simulink model "SkywalkerX8_GuidanceAndNavigation_Verification"  (R2018a)
settings: Solver=FixedStepAuto  StartTime=0.0  StopTime=375  FixedStep=0.001  RelTol=1e-3
undefined symbols (not defined in the file): DiscIntNeverNeededParam, F, Light, magnitude, MIL, SkywalkerX8
libraries: simulink_extras x13, sensors x7, simulink x3, sharedTrackingLibrary x2, aerolibwind2 x1, dspmtrx3 x1, dspsigops x1
(part 2 of 3)

== system SkywalkerX8_GuidanceAndNavigation_Verification/Autopilot Digital/Gain Scheduled Controller Phi Digital ==
  note: Since we already essentially have dphi/dt,
      | we can use it directly and create a PIDF controller
      | with PI acting on theta and the "DF" (filtered derivative)
      | simply being a filtered p
  Phi_e : Inport
  Phi : Inport  Port=2
  Va : Inport  Port=3
  p : Inport  Port=4
  DF Controller Phi : Subsystem
  PDF Controller Phi 2DOF : Subsystem
  PDF Controller Phi 2DOF Kd 2D Lookup Table : Lookup_n-D  NumberOfTableDimensions=1  BreakpointsForDimension1=SkywalkerX8.Control.Lateral.SchedulingVariables.VaArray  BreakpointsForDimension2=SkywalkerX8.Control.Longitudinal.SchedulingVariables.alphaArray  Table=SkywalkerX8.Control.Lateral.PhiController.Digital.KdPhi2DOF  InternalRulePriority=Speed  RndMeth=Simplest  InputSameDT=on
  PDF Controller Phi 2DOF Kp 2D Lookup Table : Lookup_n-D  NumberOfTableDimensions=1  BreakpointsForDimension1=SkywalkerX8.Control.Lateral.SchedulingVariables.VaArray  BreakpointsForDimension2=SkywalkerX8.Control.Longitudinal.SchedulingVariables.alphaArray  Table=SkywalkerX8.Control.Lateral.PhiController.Digital.KpPhi2DOF  InternalRulePriority=Speed  RndMeth=Simplest  InputSameDT=on
  PDF Controller Phi 2DOF N 2D Lookup Table : Lookup_n-D  NumberOfTableDimensions=1  BreakpointsForDimension1=SkywalkerX8.Control.Lateral.SchedulingVariables.VaArray  BreakpointsForDimension2=SkywalkerX8.Control.Longitudinal.SchedulingVariables.alphaArray  Table=SkywalkerX8.Control.Lateral.PhiController.Digital.NPhi2DOF  InternalRulePriority=Speed  RndMeth=Simplest  InputSameDT=on
  PI Controller Phi : Subsystem
  PIDF Controller Phi Kd 2D Lookup Table : Lookup_n-D  NumberOfTableDimensions=1  BreakpointsForDimension1=SkywalkerX8.Control.Lateral.SchedulingVariables.VaArray  BreakpointsForDimension2=SkywalkerX8.Control.Longitudinal.SchedulingVariables.alphaArray  Table=SkywalkerX8.Control.Lateral.PhiController.Digital.KdPhi  InternalRulePriority=Speed  RndMeth=Simplest  InputSameDT=on
  PIDF Controller Phi Ki 2D Lookup Table : Lookup_n-D  NumberOfTableDimensions=1  BreakpointsForDimension1=SkywalkerX8.Control.Lateral.SchedulingVariables.VaArray  BreakpointsForDimension2=SkywalkerX8.Control.Longitudinal.SchedulingVariables.alphaArray  Table=SkywalkerX8.Control.Lateral.PhiController.Digital.KiPhi  InternalRulePriority=Speed  RndMeth=Simplest  InputSameDT=on
  PIDF Controller Phi Kp 2D Lookup Table : Lookup_n-D  NumberOfTableDimensions=1  BreakpointsForDimension1=SkywalkerX8.Control.Lateral.SchedulingVariables.VaArray  BreakpointsForDimension2=SkywalkerX8.Control.Longitudinal.SchedulingVariables.alphaArray  Table=SkywalkerX8.Control.Lateral.PhiController.Digital.KpPhi  InternalRulePriority=Speed  RndMeth=Simplest  InputSameDT=on
  PIDF Controller Phi N 2D Lookup Table : Lookup_n-D  NumberOfTableDimensions=1  BreakpointsForDimension1=SkywalkerX8.Control.Lateral.SchedulingVariables.VaArray  BreakpointsForDimension2=SkywalkerX8.Control.Longitudinal.SchedulingVariables.alphaArray  Table=SkywalkerX8.Control.Lateral.PhiController.Digital.NPhi  InternalRulePriority=Speed  RndMeth=Simplest  InputSameDT=on
  Saturation : Saturate  UpperLimit=SkywalkerX8.Control.Lateral.PhiController.upperSaturationDa  LowerLimit=SkywalkerX8.Control.Lateral.PhiController.lowerSaturationDa
  Sum1 : Sum  Inputs=+++|
  Zero-Order Hold : ZeroOrderHold  SampleTime=SkywalkerX8.Control.Lateral.PhiController.Digital.SampleTime
  da : Outport
  wires:
  Va/1 -> PDF Controller Phi 2DOF Kp 2D Lookup Table/1, PDF Controller Phi 2DOF Kd 2D Lookup Table/1, PDF Controller Phi 2DOF N 2D Lookup Table/1, PIDF Controller Phi N 2D Lookup Table/1, PIDF Controller Phi Kd 2D Lookup Table/1, PIDF Controller Phi Ki 2D Lookup Table/1, PIDF Controller Phi Kp 2D Lookup Table/1
  Phi_e/1 -> PI Controller Phi/1(u)
  PIDF Controller Phi Kp 2D Lookup Table/1 -> PI Controller Phi/2(P)
  PIDF Controller Phi Ki 2D Lookup Table/1 -> PI Controller Phi/3(I)
  PI Controller Phi/1(y) -> Sum1/2
  Sum1/1 -> Saturation/1, PI Controller Phi/5(Pre-Saturation)
  p/1 -> DF Controller Phi/3(du/dt)
  DF Controller Phi/1(da*) -> Sum1/3
  PIDF Controller Phi N 2D Lookup Table/1 -> DF Controller Phi/1(N)
  PIDF Controller Phi Kd 2D Lookup Table/1 -> DF Controller Phi/2(D)
  Saturation/1 -> Zero-Order Hold/1, PI Controller Phi/4(Post-Saturation)
  PDF Controller Phi 2DOF Kp 2D Lookup Table/1 -> PDF Controller Phi 2DOF/2(P)
  PDF Controller Phi 2DOF Kd 2D Lookup Table/1 -> PDF Controller Phi 2DOF/3(D)
  PDF Controller Phi 2DOF N 2D Lookup Table/1 -> PDF Controller Phi 2DOF/4(N)
  Phi/1 -> PDF Controller Phi 2DOF/1(u)
  PDF Controller Phi 2DOF/1(y) -> Sum1/1
  Zero-Order Hold/1 -> da/1

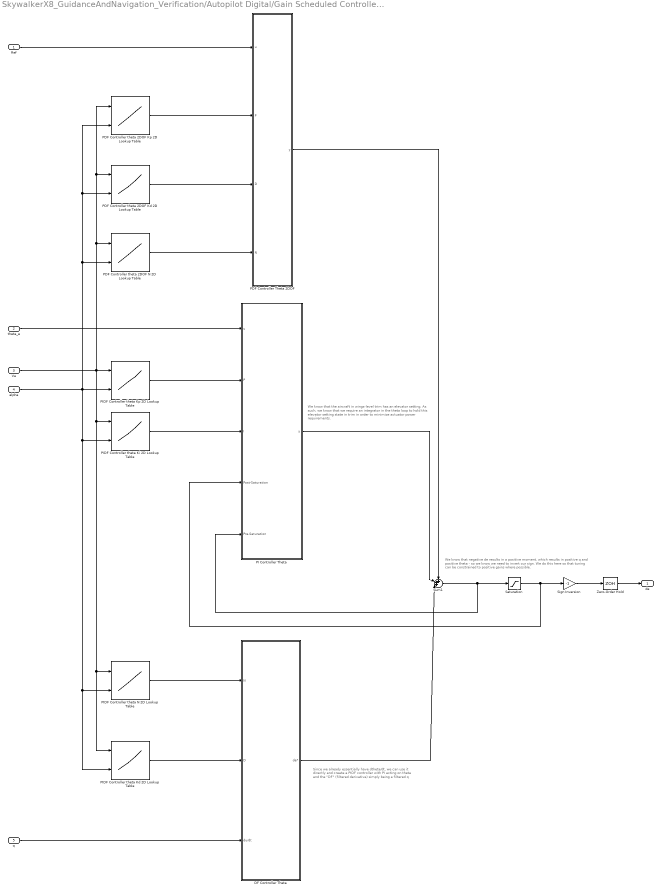
== system SkywalkerX8_GuidanceAndNavigation_Verification/Autopilot Digital/Gain Scheduled Controller Theta Digital ==
  note: Since we already essentially have dtheta/dt,
      | we can use it directly and create a PIDF controller
      | with PI acting on theta and the "DF" (filtered derivative)
      | simply being a filtered q
  note: We know that negative de results in a positive moment, which results in
      | positive q and positive theta - so we know we need to invert our sign.
      | We do this here so that tuning can be constrained to positive gains where possible.
  note: We know that the aircraft in wings-level trim has an elevator setting. As such, we know that we require an integrator in the theta loop to hold this elevator setting state in trim in order to minimize actuator power requirements.
  Ref : Inport
  theta_e : Inport  Port=2
  Va : Inport  Port=3
  alpha : Inport  Port=4
  q : Inport  Port=5
  DF Controller Theta : Subsystem
  PDF Controller Theta 2DOF : Subsystem
  PDF Controller theta 2DOF Kd 2D Lookup Table : Lookup_n-D  BreakpointsForDimension1=SkywalkerX8.Control.Longitudinal.SchedulingVariables.VaArray  BreakpointsForDimension2=SkywalkerX8.Control.Longitudinal.SchedulingVariables.alphaArray  BeginIndexSearchUsingPreviousIndexResult=on  Table=SkywalkerX8.Control.Longitudinal.thetaController.Digital.KdTheta2DOF  InternalRulePriority=Speed  RndMeth=Simplest  InputSameDT=on
  PDF Controller theta 2DOF Kp 2D Lookup Table : Lookup_n-D  BreakpointsForDimension1=SkywalkerX8.Control.Longitudinal.SchedulingVariables.VaArray  BreakpointsForDimension2=SkywalkerX8.Control.Longitudinal.SchedulingVariables.alphaArray  Table=SkywalkerX8.Control.Longitudinal.thetaController.Digital.KpTheta2DOF  InternalRulePriority=Speed  RndMeth=Simplest  InputSameDT=on
  PDF Controller theta 2DOF N 2D Lookup Table : Lookup_n-D  BreakpointsForDimension1=SkywalkerX8.Control.Longitudinal.SchedulingVariables.VaArray  BreakpointsForDimension2=SkywalkerX8.Control.Longitudinal.SchedulingVariables.alphaArray  Table=SkywalkerX8.Control.Longitudinal.thetaController.Digital.NTheta2DOF  InternalRulePriority=Speed  RndMeth=Simplest  InputSameDT=on
  PI Controller Theta : Subsystem
  PIDF Controller theta Kd 2D Lookup Table : Lookup_n-D  BreakpointsForDimension1=SkywalkerX8.Control.Longitudinal.SchedulingVariables.VaArray  BreakpointsForDimension2=SkywalkerX8.Control.Longitudinal.SchedulingVariables.alphaArray  Table=SkywalkerX8.Control.Longitudinal.thetaController.Digital.KdTheta  InternalRulePriority=Speed  RndMeth=Simplest  InputSameDT=on
  PIDF Controller theta Ki 2D Lookup Table : Lookup_n-D  BreakpointsForDimension1=SkywalkerX8.Control.Longitudinal.SchedulingVariables.VaArray  BreakpointsForDimension2=SkywalkerX8.Control.Longitudinal.SchedulingVariables.alphaArray  Table=SkywalkerX8.Control.Longitudinal.thetaController.Digital.KiTheta  InternalRulePriority=Speed  RndMeth=Simplest  InputSameDT=on
  PIDF Controller theta Kp 2D Lookup Table : Lookup_n-D  BreakpointsForDimension1=SkywalkerX8.Control.Longitudinal.SchedulingVariables.VaArray  BreakpointsForDimension2=SkywalkerX8.Control.Longitudinal.SchedulingVariables.alphaArray  Table=SkywalkerX8.Control.Longitudinal.thetaController.Digital.KpTheta  InternalRulePriority=Speed  RndMeth=Simplest  InputSameDT=on
  PIDF Controller theta N 2D Lookup Table : Lookup_n-D  BreakpointsForDimension1=SkywalkerX8.Control.Longitudinal.SchedulingVariables.VaArray  BreakpointsForDimension2=SkywalkerX8.Control.Longitudinal.SchedulingVariables.alphaArray  Table=SkywalkerX8.Control.Longitudinal.thetaController.Digital.NTheta  InternalRulePriority=Speed  RndMeth=Simplest  InputSameDT=on
  Saturation : Saturate  UpperLimit=SkywalkerX8.Control.Longitudinal.thetaController.Digital.upperSaturationNegativeDe  LowerLimit=SkywalkerX8.Control.Longitudinal.thetaController.Digital.lowerSaturationNegativeDe
  Sign Inversion : Gain  Gain=-1
  Sum1 : Sum  Inputs=+++|
  Zero-Order Hold : ZeroOrderHold  SampleTime=SkywalkerX8.Control.Longitudinal.thetaController.Digital.SampleTime
  de : Outport
  wires:
  Va/1 -> PDF Controller theta 2DOF Kd 2D Lookup Table/1, PDF Controller theta 2DOF Kp 2D Lookup Table/1, PDF Controller theta 2DOF N 2D Lookup Table/1, PIDF Controller theta N 2D Lookup Table/1, PIDF Controller theta Kd 2D Lookup Table/1, PIDF Controller theta Ki 2D Lookup Table/1, PIDF Controller theta Kp 2D Lookup Table/1
  theta_e/1 -> PI Controller Theta/1(u)
  PIDF Controller theta Kp 2D Lookup Table/1 -> PI Controller Theta/2(P)
  PIDF Controller theta Ki 2D Lookup Table/1 -> PI Controller Theta/3(I)
  alpha/1 -> PDF Controller theta 2DOF N 2D Lookup Table/2, PDF Controller theta 2DOF Kd 2D Lookup Table/2, PDF Controller theta 2DOF Kp 2D Lookup Table/2, PIDF Controller theta N 2D Lookup Table/2, PIDF Controller theta Kd 2D Lookup Table/2, PIDF Controller theta Ki 2D Lookup Table/2, PIDF Controller theta Kp 2D Lookup Table/2
  PI Controller Theta/1(y) -> Sum1/2
  Sum1/1 -> Saturation/1, PI Controller Theta/5(Pre-Saturation)
  Saturation/1 -> Sign Inversion/1, PI Controller Theta/4(Post-Saturation)
  PIDF Controller theta N 2D Lookup Table/1 -> DF Controller Theta/1(N)
  PIDF Controller theta Kd 2D Lookup Table/1 -> DF Controller Theta/2(D)
  q/1 -> DF Controller Theta/3(du/dt)
  DF Controller Theta/1(de*) -> Sum1/3
  Sign Inversion/1 -> Zero-Order Hold/1
  PDF Controller theta 2DOF Kp 2D Lookup Table/1 -> PDF Controller Theta 2DOF/2(P)
  PDF Controller theta 2DOF Kd 2D Lookup Table/1 -> PDF Controller Theta 2DOF/3(D)
  PDF Controller theta 2DOF N 2D Lookup Table/1 -> PDF Controller Theta 2DOF/4(N)
  Ref/1 -> PDF Controller Theta 2DOF/1(u)
  PDF Controller Theta 2DOF/1(y) -> Sum1/1
  Zero-Order Hold/1 -> de/1

== system SkywalkerX8_GuidanceAndNavigation_Verification/Autopilot Digital/Gain Scheduled Controller Va_dt Digital ==
  Va_e : Inport
  Va : Inport  Port=2
  TR : Inport  Port=3
  PIDF Controller Va_dt : Subsystem
  PIDF Controller Va_dt Kd Lookup Table : Lookup_n-D  NumberOfTableDimensions=1  BreakpointsForDimension1=SkywalkerX8.Control.Longitudinal.SchedulingVariables.VaArray  BreakpointsForDimension2=[1 2 3 4 5]  Table=SkywalkerX8.Control.Longitudinal.VaDtController.Digital.KdVaDt  InternalRulePriority=Speed  RndMeth=Simplest  InputSameDT=on
  PIDF Controller Va_dt Ki Lookup Table : Lookup_n-D  NumberOfTableDimensions=1  BreakpointsForDimension1=SkywalkerX8.Control.Longitudinal.SchedulingVariables.VaArray  BreakpointsForDimension2=[1 2 3 4 5]  Table=SkywalkerX8.Control.Longitudinal.VaDtController.Digital.KiVaDt  InternalRulePriority=Speed  RndMeth=Simplest  InputSameDT=on
  PIDF Controller Va_dt Kp Lookup Table : Lookup_n-D  NumberOfTableDimensions=1  BreakpointsForDimension1=SkywalkerX8.Control.Longitudinal.SchedulingVariables.VaArray  BreakpointsForDimension2=[1 2 3 4 5]  Table=SkywalkerX8.Control.Longitudinal.VaDtController.Digital.KpVaDt  InternalRulePriority=Speed  RndMeth=Simplest  InputSameDT=on
  PIDF Controller Va_dt Kt Tracking Gain Scalar : Gain  Gain=SkywalkerX8.Control.Longitudinal.VaDtController.KtScalar
  PIDF Controller Va_dt N Lookup Table : Lookup_n-D  NumberOfTableDimensions=1  BreakpointsForDimension1=SkywalkerX8.Control.Longitudinal.SchedulingVariables.VaArray  BreakpointsForDimension2=[1 2 3 4 5]  Table=SkywalkerX8.Control.Longitudinal.VaDtController.Digital.NVaDt  InternalRulePriority=Speed  RndMeth=Simplest  InputSameDT=on
  Zero-Order Hold : ZeroOrderHold  SampleTime=SkywalkerX8.Control.Longitudinal.VaDtController.Digital.SampleTime
  dt : Outport
  wires:
  Va_e/1 -> PIDF Controller Va_dt/1(u)
  PIDF Controller Va_dt/1(y) -> Zero-Order Hold/1
  PIDF Controller Va_dt Kp Lookup Table/1 -> PIDF Controller Va_dt/2(P)
  Va/1 -> PIDF Controller Va_dt Kp Lookup Table/1, PIDF Controller Va_dt Ki Lookup Table/1, PIDF Controller Va_dt N Lookup Table/1, PIDF Controller Va_dt Kd Lookup Table/1
  PIDF Controller Va_dt Ki Lookup Table/1 -> PIDF Controller Va_dt/3(I), PIDF Controller Va_dt Kt Tracking Gain Scalar/1
  PIDF Controller Va_dt Kd Lookup Table/1 -> PIDF Controller Va_dt/4(D)
  PIDF Controller Va_dt N Lookup Table/1 -> PIDF Controller Va_dt/5(N)
  TR/1 -> PIDF Controller Va_dt/7(TR)
  PIDF Controller Va_dt Kt Tracking Gain Scalar/1 -> PIDF Controller Va_dt/6(Kt)
  Zero-Order Hold/1 -> dt/1

== system SkywalkerX8_GuidanceAndNavigation_Verification/Autopilot Digital/Gain Scheduled Controller Va_theta Digital ==
  note: We know that negative theta results in positive Va (as we'll start losing altitude)
      | and vice versa as we gain altitude. In order to keep our controller gains positive
      |  we do the sign inversion seperately.
  note: Because we sign invert the output, we need to sign invert the tracking
      | value
  Va_e : Inport
  Va : Inport  Port=2
  alpha : Inport  Port=3
  TR : Inport  Port=4
  PIDF Controller Va_theta : Subsystem
  PIDF Controller Va_theta Kd 2D Lookup Table : Lookup_n-D  BreakpointsForDimension1=SkywalkerX8.Control.Longitudinal.SchedulingVariables.VaArray  BreakpointsForDimension2=SkywalkerX8.Control.Longitudinal.SchedulingVariables.alphaArray  Table=SkywalkerX8.Control.Longitudinal.VaThetaController.Digital.KdVaTheta  InternalRulePriority=Speed  RndMeth=Simplest  InputSameDT=on
  PIDF Controller Va_theta Ki 2D Lookup Table : Lookup_n-D  BreakpointsForDimension1=SkywalkerX8.Control.Longitudinal.SchedulingVariables.VaArray  BreakpointsForDimension2=SkywalkerX8.Control.Longitudinal.SchedulingVariables.alphaArray  Table=SkywalkerX8.Control.Longitudinal.VaThetaController.Digital.KiVaTheta  InternalRulePriority=Speed  RndMeth=Simplest  InputSameDT=on
  PIDF Controller Va_theta Kp 2D Lookup Table : Lookup_n-D  BreakpointsForDimension1=SkywalkerX8.Control.Longitudinal.SchedulingVariables.VaArray  BreakpointsForDimension2=SkywalkerX8.Control.Longitudinal.SchedulingVariables.alphaArray  Table=SkywalkerX8.Control.Longitudinal.VaThetaController.Digital.KpVaTheta  InternalRulePriority=Speed  RndMeth=Simplest  InputSameDT=on
  PIDF Controller Va_theta Kt Tracking Gain Scalar : Gain  Gain=SkywalkerX8.Control.Longitudinal.VaThetaController.KtScalar
  PIDF Controller Va_theta N 2D Lookup Table : Lookup_n-D  BreakpointsForDimension1=SkywalkerX8.Control.Longitudinal.SchedulingVariables.VaArray  BreakpointsForDimension2=SkywalkerX8.Control.Longitudinal.SchedulingVariables.alphaArray  Table=SkywalkerX8.Control.Longitudinal.VaThetaController.Digital.NVaTheta  InternalRulePriority=Speed  RndMeth=Simplest  InputSameDT=on
  Sign Inversion : Gain  Gain=-1
  Tracking Sign Inversion : Gain  Gain=-1
  Zero-Order Hold : ZeroOrderHold  SampleTime=SkywalkerX8.Control.Longitudinal.altController.Digital.SampleTime
  theta_c_Va : Outport
  wires:
  Va_e/1 -> PIDF Controller Va_theta/1(u)
  PIDF Controller Va_theta/1(y) -> Sign Inversion/1
  PIDF Controller Va_theta Kp 2D Lookup Table/1 -> PIDF Controller Va_theta/2(P)
  Va/1 -> PIDF Controller Va_theta Kp 2D Lookup Table/1, PIDF Controller Va_theta Ki 2D Lookup Table/1, PIDF Controller Va_theta N 2D Lookup Table/1, PIDF Controller Va_theta Kd 2D Lookup Table/1
  PIDF Controller Va_theta Ki 2D Lookup Table/1 -> PIDF Controller Va_theta/3(I), PIDF Controller Va_theta Kt Tracking Gain Scalar/1
  PIDF Controller Va_theta Kd 2D Lookup Table/1 -> PIDF Controller Va_theta/4(D)
  PIDF Controller Va_theta N 2D Lookup Table/1 -> PIDF Controller Va_theta/5(N)
  alpha/1 -> PIDF Controller Va_theta Kp 2D Lookup Table/2, PIDF Controller Va_theta Ki 2D Lookup Table/2, PIDF Controller Va_theta N 2D Lookup Table/2, PIDF Controller Va_theta Kd 2D Lookup Table/2
  Sign Inversion/1 -> Zero-Order Hold/1
  TR/1 -> Tracking Sign Inversion/1
  PIDF Controller Va_theta Kt Tracking Gain Scalar/1 -> PIDF Controller Va_theta/6(Kt)
  Tracking Sign Inversion/1 -> PIDF Controller Va_theta/7(TR)
  Zero-Order Hold/1 -> theta_c_Va/1

== system SkywalkerX8_GuidanceAndNavigation_Verification/Autopilot Digital/Gain Scheduled Controller h_theta Digital ==
  note: We know that wings-level trim has the aircraft with a pitch angle. As such,
      | we know that at a minimum this controller has to be a PI controller, because otherwise
      | we have no state to hold the required steady state theta command.
  h_e : Inport
  TR : Inport  Port=2
  Kd : Constant  Value=SkywalkerX8.Control.Longitudinal.altController.Digital.KdAlt(5, 3)
  Ki : Constant  Value=SkywalkerX8.Control.Longitudinal.altController.Digital.KiAlt(5, 3)
  Kp : Constant  Value=SkywalkerX8.Control.Longitudinal.altController.Digital.KpAlt(5, 3)
  Kt : Constant  Value=SkywalkerX8.Control.Longitudinal.altController.KtScalar*SkywalkerX8.Control.Longitudinal.altController.Digital.KiAlt(5, 3)
  N : Constant  Value=SkywalkerX8.Control.Longitudinal.altController.Digital.NAlt(5, 3)
  PIDF Controller h_theta : Subsystem
  Zero-Order Hold : ZeroOrderHold  SampleTime=SkywalkerX8.Control.Longitudinal.altController.Digital.SampleTime
  theta_c_h : Outport
  wires:
  Kp/1 -> PIDF Controller h_theta/2(P)
  h_e/1 -> PIDF Controller h_theta/1(u)
  Kd/1 -> PIDF Controller h_theta/4(D)
  N/1 -> PIDF Controller h_theta/5(N)
  PIDF Controller h_theta/1(y) -> Zero-Order Hold/1
  TR/1 -> PIDF Controller h_theta/7(TR)
  Ki/1 -> PIDF Controller h_theta/3(I)
  Kt/1 -> PIDF Controller h_theta/6(Kt)
  Zero-Order Hold/1 -> theta_c_h/1

== system SkywalkerX8_GuidanceAndNavigation_Verification/Autopilot Digital/h Rate Limiter Dynamic ==
  note: U(k)
  note: Y(k)
  up : Inport
  u : Inport  Port=2
  lo : Inport  Port=3
  Delay Input2 : UnitDelay  Description=Store in Global RAM  DisableCoverage=on  InitialCondition=initOutput  SampleTime=-1
  Difference Inputs1 : Sum  Description=Add in CPU  DisableCoverage=on  Inputs=+-  OutDataTypeStr=Inherit: Inherit via back propagation
  Difference Inputs2 : Sum  Description=Add in CPU  OutDataTypeStr=Inherit: Inherit via back propagation
  FixPt Data Type Duplicate : DataTypeDuplicate  DisableCoverage=on  NumInputPorts=7
  Saturation Dynamic : simulink/Discontinuities/Saturation Dynamic  OutMin=[]  OutMax=[]  OutDataTypeStr=Inherit: Same as second input  OutDataType=fixdt(1, 16)  OutScaling=2^-10  DoSatur=off
  delta fall limit : Product  DisableCoverage=on  Inputs=**  OutDataTypeStr=Inherit: Inherit via back propagation  SaturateOnIntegerOverflow=on
  delta rise limit : Product  DisableCoverage=on  Inputs=**  OutDataTypeStr=Inherit: Inherit via back propagation  SaturateOnIntegerOverflow=on
  sample time : SampleTimeMath  DisableCoverage=on  TsampMathOp=Ts Only  weightValue=1
  Y : Outport  InitialOutput=0
  wires:
  Delay Input2/1 -> Difference Inputs1/2, FixPt Data Type Duplicate/2, Difference Inputs2/2  "Y(k-1)"
  Difference Inputs1/1 -> FixPt Data Type Duplicate/4, Saturation Dynamic/2  "( U(k) - Y(k-1) )"
  Difference Inputs2/1 -> Y/1, Delay Input2/1, FixPt Data Type Duplicate/1
  u/1 -> Difference Inputs1/1, FixPt Data Type Duplicate/5, sample time/1
  delta fall limit/1 -> FixPt Data Type Duplicate/3, Saturation Dynamic/3
  sample time/1 -> delta fall limit/2, delta rise limit/2
  Saturation Dynamic/1 -> Difference Inputs2/1, FixPt Data Type Duplicate/7
  delta rise limit/1 -> FixPt Data Type Duplicate/6, Saturation Dynamic/1
  lo/1 -> delta fall limit/1
  up/1 -> delta rise limit/1

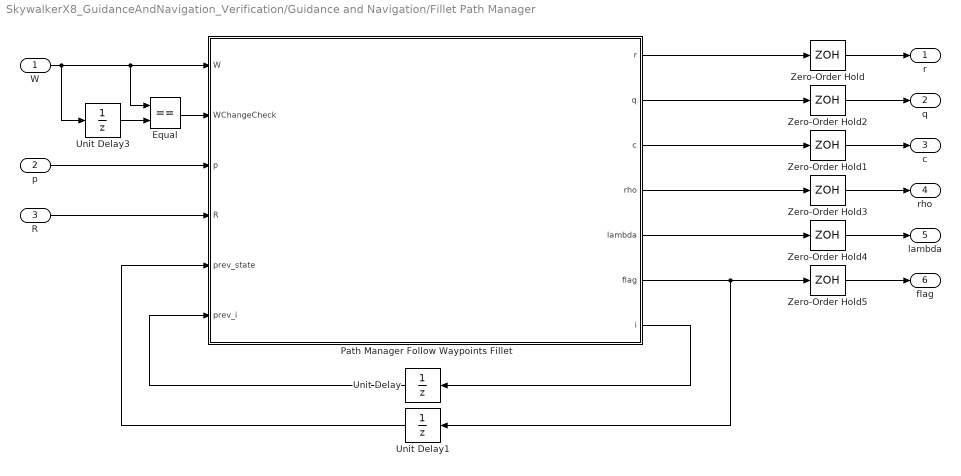
== system SkywalkerX8_GuidanceAndNavigation_Verification/Guidance and Navigation/Fillet Path Manager ==
  W : Inport
  p : Inport  Port=2
  R : Inport  Port=3
  Equal : RelationalOperator  Operator===  OutDataTypeStr=boolean  RndMeth=Simplest
  Path Manager Follow Waypoints Fillet : MATLAB Function  TreatAsAtomicUnit=on
  Unit Delay : UnitDelay  InitialCondition=2  SampleTime=SampleTime
  Unit Delay1 : UnitDelay  InitialCondition=1  SampleTime=SampleTime
  Unit Delay3 : UnitDelay  InitialCondition=SkywalkerX8.Test.Waypoints  SampleTime=SampleTime
  Zero-Order Hold{,1..5} (6 alike) : ZeroOrderHold  SampleTime=SampleTime
  r : Outport
  q : Outport  Port=2
  c : Outport  Port=3
  rho : Outport  Port=4
  lambda : Outport  Port=5
  flag : Outport  Port=6
  wires:
  Path Manager Follow Waypoints Fillet/2(q) -> Zero-Order Hold2/1
  Path Manager Follow Waypoints Fillet/6(flag) -> Zero-Order Hold5/1, Unit Delay1/1
  W/1 -> Unit Delay3/1, Equal/1, Path Manager Follow Waypoints Fillet/1(W)
  Unit Delay/1 -> Path Manager Follow Waypoints Fillet/6(prev_i)
  Path Manager Follow Waypoints Fillet/7(i) -> Unit Delay/1
  Path Manager Follow Waypoints Fillet/3(c) -> Zero-Order Hold1/1
  p/1 -> Path Manager Follow Waypoints Fillet/3(p)
  Path Manager Follow Waypoints Fillet/4(rho) -> Zero-Order Hold3/1
  Path Manager Follow Waypoints Fillet/1(r) -> Zero-Order Hold/1
  Unit Delay1/1 -> Path Manager Follow Waypoints Fillet/5(prev_state)
  R/1 -> Path Manager Follow Waypoints Fillet/4(R)
  Zero-Order Hold/1 -> r/1
  Zero-Order Hold1/1 -> c/1
  Zero-Order Hold2/1 -> q/1
  Zero-Order Hold3/1 -> rho/1
  Zero-Order Hold4/1 -> lambda/1
  Zero-Order Hold5/1 -> flag/1
  Path Manager Follow Waypoints Fillet/5(lambda) -> Zero-Order Hold4/1
  Unit Delay3/1 -> Equal/2
  Equal/1 -> Path Manager Follow Waypoints Fillet/2(WChangeCheck)

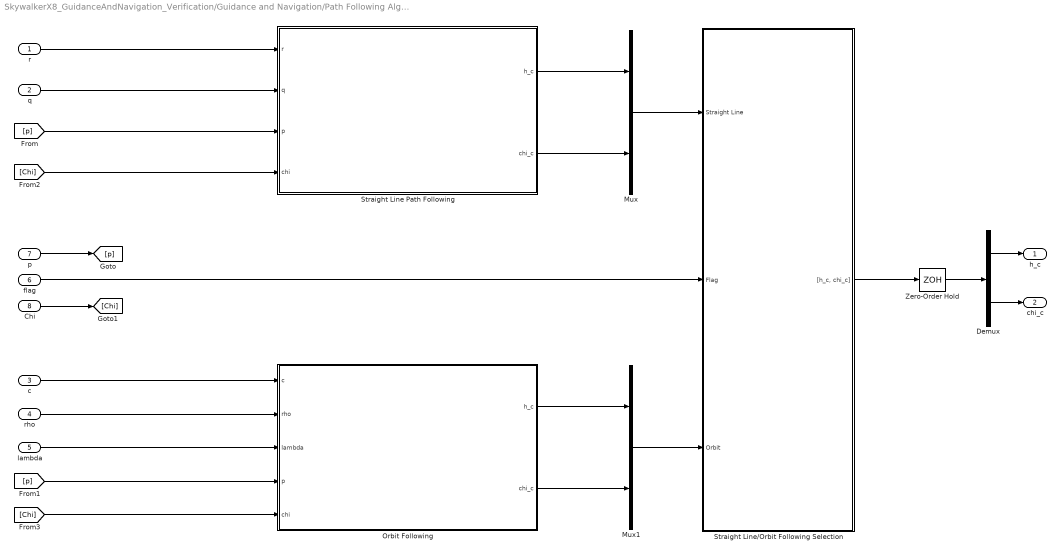
== system SkywalkerX8_GuidanceAndNavigation_Verification/Guidance and Navigation/Path Following Algorithm ==
  r : Inport
  q : Inport  Port=2
  c : Inport  Port=3
  rho : Inport  Port=4
  lambda : Inport  Port=5
  flag : Inport  Port=6
  p : Inport  Port=7
  Chi : Inport  Port=8
  Demux : Demux  Outputs=2
  Mux : Mux  Inputs=2
  Mux1 : Mux  Inputs=2
  Orbit Following : MATLAB Function  TreatAsAtomicUnit=on  mask{korbit=korbit}
      mask prompts: korbit "kOrbit (Unitless)"
  Straight Line Path Following : MATLAB Function  TreatAsAtomicUnit=on  mask{chi_inf=ChiInf, kpath=kpath}
      mask prompts: chi_inf "Chi_inf (rad)"; kpath "kPath (Unitless)"
  Straight Line/Orbit Following Selection : Subsystem
      mask Display:
      | port_label('input', 1, '[h_c, \chi_c]_{Straight Line} (m, rad)', 'texMode', 'On')
      | port_label('input', 2, 'Flag (Unitless)', 'texMode', 'On')
      | port_label('input', 3, '[h_c, \chi_c]_{Orbit Following} (m, rad)', 'texMode', 'On')
      | 
      | port_label('output', 1, '[h_c, \chi_c] (m, rad)', 'texMode', 'On')
  Zero-Order Hold : ZeroOrderHold  SampleTime=SampleTime
  h_c : Outport
  chi_c : Outport  Port=2
  wires:
  [Chi] -> Orbit Following/5(chi)
  rho/1 -> Orbit Following/2(rho)
  r/1 -> Straight Line Path Following/1(r)
  Orbit Following/2(chi_c) -> Mux1/2
  q/1 -> Straight Line Path Following/2(q)
  p/1 -> [p]
  lambda/1 -> Orbit Following/3(lambda)
  Orbit Following/1(h_c) -> Mux1/1
  Straight Line/Orbit Following Selection/1("[h_c, chi_c]") -> Zero-Order Hold/1
  Mux/1 -> Straight Line/Orbit Following Selection/1(Straight Line)
  c/1 -> Orbit Following/1(c)
  Mux1/1 -> Straight Line/Orbit Following Selection/3(Orbit)
  Straight Line Path Following/2(chi_c) -> Mux/2
  [Chi] -> Straight Line Path Following/4(chi)
  flag/1 -> Straight Line/Orbit Following Selection/2(Flag)
  [p] -> Straight Line Path Following/3(p)
  Straight Line Path Following/1(h_c) -> Mux/1
  Chi/1 -> [Chi]
  [p] -> Orbit Following/4(p)
  Zero-Order Hold/1 -> Demux/1
  Demux/1 -> h_c/1
  Demux/2 -> chi_c/1

== system SkywalkerX8_GuidanceAndNavigation_Verification/Sensor Suite/9-Axis MEMS IMU ==
  ainertial : Inport
  PhiThetaPsi : Inport  Port=2
  pqr : Inport  Port=3
  3-Axis Accelerometer : sensors/3-Axis Accelerometer  g=SkywalkerX8.System.Gravity  SampleTime=SkywalkerX8.Sensors.IMU.Accelerometer.SampleTime  accelXNoiseDensity=SkywalkerX8.Sensors.IMU.Accelerometer.X.NoiseDensity  accelYNoiseDensity=SkywalkerX8.Sensors.IMU.Accelerometer.Y.NoiseDensity  accelZNoiseDensity=SkywalkerX8.Sensors.IMU.Accelerometer.Z.NoiseDensity  accelXBandwidthHz=SkywalkerX8.Sensors.IMU.Accelerometer.X.BandwidthHz  accelYBandwidthHz=SkywalkerX8.Sensors.IMU.Accelerometer.Y.BandwidthHz  accelZBandwidthHz=SkywalkerX8.Sensors.IMU.Accelerometer.Z.BandwidthHz  accelXInit=SkywalkerX8.Sensors.IMU.Accelerometer.X.InitialCondition  accelYInit=SkywalkerX8.Sensors.IMU.Accelerometer.Y.InitialCondition  accelZInit=SkywalkerX8.Sensors.IMU.Accelerometer.Z.InitialCondition  accelXUpperSaturation=SkywalkerX8.Sensors.IMU.Accelerometer.X.UpperSat  accelXLowerSaturation=SkywalkerX8.Sensors.IMU.Accelerometer.X.LowerSat  accelYUpperSaturation=SkywalkerX8.Sensors.IMU.Accelerometer.Y.UpperSat  accelYLowerSaturation=SkywalkerX8.Sensors.IMU.Accelerometer.Y.LowerSat  accelZUpperSaturation=SkywalkerX8.Sensors.IMU.Accelerometer.Z.UpperSat  accelZLowerSaturation=SkywalkerX8.Sensors.IMU.Accelerometer.Z.LowerSat  accelXResolution=SkywalkerX8.Sensors.IMU.Accelerometer.X.Resolution  accelYResolution=SkywalkerX8.Sensors.IMU.Accelerometer.Y.Resolution  accelZResolution=SkywalkerX8.Sensors.IMU.Accelerometer.Z.Resolution
  3-Axis MEMS Gyroscope : sensors/3-Axis MEMS Gyroscope  SampleTime=SkywalkerX8.Sensors.IMU.Gyroscope.SampleTime  gyroXNoiseDensity=SkywalkerX8.Sensors.IMU.Gyroscope.X.NoiseDensity  gyroYNoiseDensity=SkywalkerX8.Sensors.IMU.Gyroscope.Y.NoiseDensity  gyroZNoiseDensity=SkywalkerX8.Sensors.IMU.Gyroscope.Z.NoiseDensity  gyroXBandwidthHz=SkywalkerX8.Sensors.IMU.Gyroscope.X.BandwidthHz  gyroYBandwidthHz=SkywalkerX8.Sensors.IMU.Gyroscope.Y.BandwidthHz  gyroZBandwidthHz=SkywalkerX8.Sensors.IMU.Gyroscope.Z.BandwidthHz  gyroXInit=SkywalkerX8.Sensors.IMU.Gyroscope.X.InitialCondition  gyroYInit=SkywalkerX8.Sensors.IMU.Gyroscope.Y.InitialCondition  gyroZInit=SkywalkerX8.Sensors.IMU.Gyroscope.Z.InitialCondition  gyroXUpperSaturation=SkywalkerX8.Sensors.IMU.Gyroscope.X.UpperSat  gyroXLowerSaturation=SkywalkerX8.Sensors.IMU.Gyroscope.X.LowerSat  gyroYUpperSaturation=SkywalkerX8.Sensors.IMU.Gyroscope.Y.UpperSat  gyroYLowerSaturation=SkywalkerX8.Sensors.IMU.Gyroscope.Y.LowerSat  gyroZUpperSaturation=SkywalkerX8.Sensors.IMU.Gyroscope.Z.UpperSat  gyroZLowerSaturation=SkywalkerX8.Sensors.IMU.Gyroscope.Z.LowerSat  gyroXResolution=SkywalkerX8.Sensors.IMU.Gyroscope.X.Resolution  gyroYResolution=SkywalkerX8.Sensors.IMU.Gyroscope.Y.Resolution  gyroZResolution=SkywalkerX8.Sensors.IMU.Gyroscope.Z.Resolution
  3-Axis Magnetometer Compass : sensors/3-Axis Magnetometer Compass  SampleTime=SkywalkerX8.Sensors.IMU.Compass.SampleTime  headingNoiseDensity=SkywalkerX8.Sensors.IMU.Compass.NoiseDensity  headingBandwidthHz=SkywalkerX8.Sensors.IMU.Compass.BandwidthHz  headingInit=SkywalkerX8.Sensors.IMU.Compass.InitialCondition  headingUpperSaturation=SkywalkerX8.Sensors.IMU.Compass.UpperSat  headingLowerSaturation=SkywalkerX8.Sensors.IMU.Compass.LowerSat  headingResolution=SkywalkerX8.Sensors.IMU.Compass.Resolution
  Selector : Selector  InputPortWidth=3  IndexOptions=Index vector (dialog)  Indices=3  OutputSizes=1
  yAccelerometer : Outport
  yGyro : Outport  Port=2
  yPsi : Outport  Port=3
  wires:
  ainertial/1 -> 3-Axis Accelerometer/1
  PhiThetaPsi/1 -> 3-Axis Accelerometer/2, Selector/1
  Selector/1 -> 3-Axis Magnetometer Compass/1
  pqr/1 -> 3-Axis MEMS Gyroscope/1
  3-Axis MEMS Gyroscope/1 -> yGyro/1
  3-Axis Accelerometer/1 -> yAccelerometer/1
  3-Axis Magnetometer Compass/1 -> yPsi/1

== system SkywalkerX8_GuidanceAndNavigation_Verification/State Estimation/Attitude Estimation Extended Kalman Filter with Filtering ==
  u : Inport
  y : Inport  Port=2
  Attitude Estimation Extended Kalman Filter : Subsystem
      mask Display:
      | port_label('input', 1, '{\bf u} = [p, q, r, V_a, \alpha]', 'texMode', 'On')
      | port_label('input', 2, '{\bf y} = [a_x, a_y, a_z]', 'texMode', 'On')
      | 
      | port_label('output', 1, '{\bf x_{est}} = [\Phi, \theta]', 'texMode', 'On')
  xest : Outport
  wires:
  y/1 -> Attitude Estimation Extended Kalman Filter/2(y)
  Attitude Estimation Extended Kalman Filter/1(xhat) -> xest/1
  u/1 -> Attitude Estimation Extended Kalman Filter/1(u)

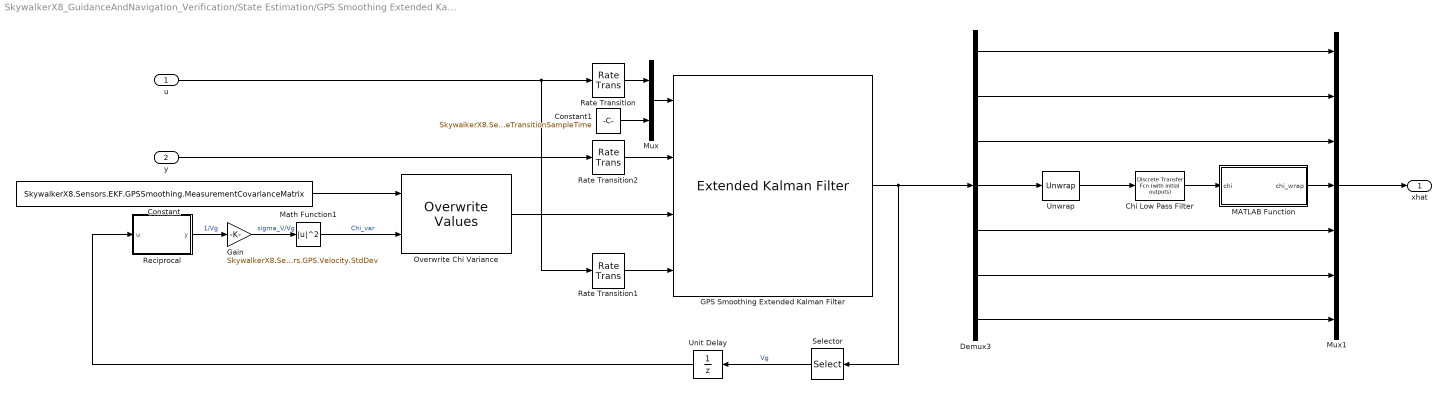
== system SkywalkerX8_GuidanceAndNavigation_Verification/State Estimation/GPS Smoothing Extended Kalman Filter ==
  u : Inport  PortDimensions=5
  y : Inport  Port=2  PortDimensions=6
  Chi Low Pass Filter : simulink_extras/Additional Discrete/Discrete Transfer Fcn (with initial outputs)  N=cell2mat(SkywalkerX8.Sensors.EKF.GPSSmoothing.Filters.ChiFilter.TFDigital.Numerator)  D=cell2mat(SkywalkerX8.Sensors.EKF.GPSSmoothing.Filters.ChiFilter.TFDigital.Denominator)  U0=SkywalkerX8.Sensors.EKF.GPSSmoothing.Filters.ChiFilter.InitialCondition  Y0=SkywalkerX8.Sensors.EKF.GPSSmoothing.Filters.ChiFilter.InitialCondition  TS=SkywalkerX8.Sensors.EKF.GPSSmoothing.Filters.ChiFilter.SampleTime
      settings: SourceProductName=Simulink  SourceProductBaseCode=SL
  Constant : Constant  Value=SkywalkerX8.Sensors.EKF.GPSSmoothing.MeasurementCovarianceMatrix
  Constant1 : Constant  Value=SkywalkerX8.Sensors.EKF.GPSSmoothing.StateTransitionSampleTime
  Demux3 : Demux  Outputs=7
  GPS Smoothing Extended Kalman Filter : sharedTrackingLibrary/Extended Kalman Filter  StateTransitionFcn=GPSSmoothingTransitionEstimate  HasStateTransitionJacobianFcn=on  StateTransitionJacobianFcn=GPSSmoothingTransitionEstimate_Jacobian  HasAdditiveProcessNoise=Additive  ProcessNoise=SkywalkerX8.Sensors.EKF.GPSSmoothing.ProcessCovarianceMatrix  HasTimeVaryingProcessNoise=off  HasStateTransitionFcnExtraArgument=1  InitialState=SkywalkerX8.Sensors.EKF.GPSSmoothing.InitialState  InitialStateCovariance=SkywalkerX8.Sensors.EKF.GPSSmoothing.InitialStateCovarianceMatrix  MeasurementFcn1=GPSSmoothingMeasurementEstimate  HasMeasurementJacobianFcn1=on  MeasurementJacobianFcn1=GPSSmoothingMeasurementEstimate_Jacobian  HasMeasurementEnablePort1=off  HasAdditiveMeasurementNoise1=Additive  MeasurementNoise1=SkywalkerX8.Sensors.EKF.GPSSmoothing.MeasurementCovarianceMatrix  HasTimeVaryingMeasurementNoise1=on  HasMeasurementFcnExtraArgument1=1  MeasurementFcn2=myMeasurementFcn  HasMeasurementJacobianFcn2=off  HasMeasurementEnablePort2=off  HasAdditiveMeasurementNoise2=Additive  MeasurementNoise2=1  HasTimeVaryingMeasurementNoise2=off  HasMeasurementFcnExtraArgument2=0  MeasurementFcn3=myMeasurementFcn  HasMeasurementJacobianFcn3=off  HasMeasurementEnablePort3=off  HasAdditiveMeasurementNoise3=Additive  MeasurementNoise3=1  HasTimeVaryingMeasurementNoise3=off  HasMeasurementFcnExtraArgument3=0  MeasurementFcn4=myMeasurementFcn  HasMeasurementJacobianFcn4=off  HasMeasurementEnablePort4=off  HasAdditiveMeasurementNoise4=Additive  MeasurementNoise4=1  HasTimeVaryingMeasurementNoise4=off  HasMeasurementFcnExtraArgument4=0  MeasurementFcn5=myMeasurementFcn  HasMeasurementJacobianFcn5=off  HasMeasurementEnablePort5=off  HasAdditiveMeasurementNoise5=Additive  MeasurementNoise5=1  HasTimeVaryingMeasurementNoise5=off  HasMeasurementFcnExtraArgument5=0  EnableMultirate=on  StateTransitionFcnSampleTime=SkywalkerX8.Sensors.EKF.GPSSmoothing.StateTransitionSampleTime  MeasurementFcn1SampleTime=SkywalkerX8.Sensors.EKF.GPSSmoothing.MeasurementSampleTime  MeasurementFcn2SampleTime=1  MeasurementFcn3SampleTime=1  MeasurementFcn4SampleTime=1  MeasurementFcn5SampleTime=1  UseCurrentEstimator=on  OutputStateCovariance=off  DataType=double  SampleTime=SkywalkerX8.Sensors.EKF.GPSSmoothing.SampleTime  NumberOfMeasurements=1
      settings: SourceProductName=Control System Toolbox  SourceProductBaseCode=CT
  Gain : Gain  Gain=SkywalkerX8.Sensors.GPS.Velocity.StdDev
  MATLAB Function : MATLAB Function  TreatAsAtomicUnit=on
  Math Function1 : Math  Operator=magnitude^2  SaturateOnIntegerOverflow=on
  Mux : Mux  Inputs=2
  Mux1 : Mux  Inputs=7
  Overwrite Chi Variance : dspmtrx3/Overwrite Values  OverWriteDiag=Submatrix  valFrom2ndIP=Second input port  ConstValue=0  RowSpan=One row  RowStartMode=Index  RowStartIndex=4  RowEndMode=Last  RowEndIndex=1  ColSpan=One column  ColStartMode=First  ColStartIndex=1  ColEndMode=Last  ColEndIndex=1  DiagSpan=Range of elements  DiagStartMode=Index  DiagStartIndex=2  DiagEndMode=Index  DiagEndIndex=4
      settings: SourceProductName=DSP System Toolbox  SourceProductBaseCode=DS
  Rate Transition : RateTransition  InitialCondition=SkywalkerX8.Sensors.EKF.GPSSmoothing.InitialInput  OutPortSampleTime=SkywalkerX8.Sensors.EKF.GPSSmoothing.StateTransitionSampleTime
  Rate Transition1 : RateTransition  InitialCondition=SkywalkerX8.Sensors.EKF.GPSSmoothing.InitialInput  OutPortSampleTime=SkywalkerX8.Sensors.EKF.GPSSmoothing.MeasurementSampleTime
  Rate Transition2 : RateTransition  InitialCondition=SkywalkerX8.Sensors.EKF.GPSSmoothing.InitialMeasurement  OutPortSampleTime=SkywalkerX8.Sensors.EKF.GPSSmoothing.MeasurementSampleTime
  Reciprocal : MATLAB Function  TreatAsAtomicUnit=on
  Selector : Selector  InputPortWidth=7  IndexOptions=Index vector (dialog)  Indices=3  OutputSizes=1
  Unit Delay : UnitDelay  InitialCondition=SkywalkerX8.Sensors.EKF.GPSSmoothing.InitialState(3)  SampleTime=SkywalkerX8.Sensors.EKF.GPSSmoothing.MeasurementSampleTime
  Unwrap : dspsigops/Unwrap  tol=pi  InputProcessing=Columns as channels (frame based)  running=off
  xhat : Outport
  wires:
  y/1 -> Rate Transition2/1
  GPS Smoothing Extended Kalman Filter/1 -> Demux3/1, Selector/1
  Reciprocal/1(y) -> Gain/1  "1/Vg"
  Gain/1 -> Math Function1/1  "sigma_V/Vg"
  Math Function1/1 -> Overwrite Chi Variance/2  "Chi_var"
  Constant/1 -> Overwrite Chi Variance/1
  Overwrite Chi Variance/1 -> GPS Smoothing Extended Kalman Filter/3
  u/1 -> Rate Transition1/1, Rate Transition/1
  Selector/1 -> Unit Delay/1  "Vg"
  Unit Delay/1 -> Reciprocal/1(u)
  Rate Transition1/1 -> GPS Smoothing Extended Kalman Filter/4
  Rate Transition2/1 -> GPS Smoothing Extended Kalman Filter/2
  Rate Transition/1 -> Mux/1
  Mux/1 -> GPS Smoothing Extended Kalman Filter/1
  Constant1/1 -> Mux/2
  Demux3/1 -> Mux1/1
  Demux3/2 -> Mux1/2
  Demux3/3 -> Mux1/3
  Mux1/1 -> xhat/1
  Demux3/4 -> Unwrap/1
  Chi Low Pass Filter/1 -> MATLAB Function/1(chi)
  Demux3/5 -> Mux1/5
  Demux3/6 -> Mux1/6
  Demux3/7 -> Mux1/7
  Unwrap/1 -> Chi Low Pass Filter/1
  MATLAB Function/1(chi_wrap) -> Mux1/4

== system SkywalkerX8_GuidanceAndNavigation_Verification/Autopilot Digital/Gain Scheduled Controller Chi Digital/PIDF Controller Va_theta ==
  u : Inport
  P : Inport  Port=2
  I : Inport  Port=3
  Post-Saturation : Inport  Port=4
  Pre-Saturation : Inport  Port=5
  Clamp Switch : Switch  Criteria=u2 ~= 0
  Clamping circuit : Subsystem
  Constant : Constant  Value=0
  Discrete-Time Integrator : DiscreteIntegrator  IntegratorMethod=Integration: Trapezoidal  InitialCondition=SkywalkerX8.InitialConditions.PhiThetaPsi(1)  SampleTime=SkywalkerX8.Control.Lateral.ChiController.Digital.SampleTime  ICPrevOutput=DiscIntNeverNeededParam  ICPrevScaledInput=DiscIntNeverNeededParam
  IOut : Product  DisableCoverage=on
  POut : Product
  Sum2 : Sum  Inputs=++|
  y : Outport  InitialOutput=0
  wires:
  Sum2/1 -> y/1
  POut/1 -> Sum2/1
  u/1 -> POut/2, IOut/2  "u"
  Clamp Switch/1 -> Discrete-Time Integrator/1
  Discrete-Time Integrator/1 -> Sum2/2
  Constant/1 -> Clamp Switch/1
  I/1 -> IOut/1  "Ki"
  IOut/1 -> Clamp Switch/3  "IOut"
  Clamping circuit/1(Clamp) -> Clamp Switch/2
  P/1 -> POut/1
  Pre-Saturation/1 -> Clamping circuit/1(preSat)
  Post-Saturation/1 -> Clamping circuit/2(postSat)

== system SkywalkerX8_GuidanceAndNavigation_Verification/Autopilot Digital/Gain Scheduled Controller Phi Digital/DF Controller Phi ==
  N : Inport
  D : Inport  Port=2
  du/dt : Inport  Port=3
  Discrete-Time Integrator : DiscreteIntegrator  SampleTime=SkywalkerX8.Control.Lateral.PhiController.Digital.SampleTime  ICPrevOutput=DiscIntNeverNeededParam  ICPrevScaledInput=DiscIntNeverNeededParam
  Product : Product
  Product1 : Product
  Sum : Sum  Inputs=|+-
  da* : Outport
  wires:
  Discrete-Time Integrator/1 -> da*/1, Sum/2  "da*"
  Product1/1 -> Discrete-Time Integrator/1  "Nda*_e"
  du/dt/1 -> Product/2
  D/1 -> Product/1
  Sum/1 -> Product1/2  "da*_e"
  N/1 -> Product1/1
  Product/1 -> Sum/1

== system SkywalkerX8_GuidanceAndNavigation_Verification/Autopilot Digital/Gain Scheduled Controller Phi Digital/PDF Controller Phi 2DOF ==
  u : Inport
  P : Inport  Port=2
  D : Inport  Port=3
  N : Inport  Port=4
  Discrete-Time Integrator : DiscreteIntegrator  SampleTime=SkywalkerX8.Control.Lateral.PhiController.Digital.SampleTime  ICPrevOutput=DiscIntNeverNeededParam  ICPrevScaledInput=DiscIntNeverNeededParam
  POut : Product
  Product : Product
  Product1 : Product
  Sum : Sum  Inputs=|+-
  Sum2 : Sum
  y : Outport  InitialOutput=0
  wires:
  Sum2/1 -> y/1
  N/1 -> Product1/1
  Product1/1 -> Discrete-Time Integrator/1, Sum2/2
  Sum/1 -> Product1/2
  POut/1 -> Sum2/1
  D/1 -> Product/2
  u/1 -> Product/1, POut/2  "u"
  Discrete-Time Integrator/1 -> Sum/2
  Product/1 -> Sum/1
  P/1 -> POut/1

== system SkywalkerX8_GuidanceAndNavigation_Verification/Autopilot Digital/Gain Scheduled Controller Phi Digital/PI Controller Phi ==
  u : Inport
  P : Inport  Port=2
  I : Inport  Port=3
  Post-Saturation : Inport  Port=4
  Pre-Saturation : Inport  Port=5
  Clamp Switch : Switch  Criteria=u2 ~= 0
  Clamping circuit : Subsystem
  Constant : Constant  Value=0
  Discrete-Time Integrator : DiscreteIntegrator  IntegratorMethod=Integration: Trapezoidal  InitialCondition=SkywalkerX8.InitialConditions.da  SampleTime=SkywalkerX8.Control.Lateral.PhiController.Digital.SampleTime  ICPrevOutput=DiscIntNeverNeededParam  ICPrevScaledInput=DiscIntNeverNeededParam
  IOut : Product  DisableCoverage=on
  POut : Product
  Sum2 : Sum  Inputs=|++
  y : Outport  InitialOutput=0
  wires:
  IOut/1 -> Clamp Switch/3
  Clamp Switch/1 -> Discrete-Time Integrator/1
  Sum2/1 -> y/1
  Pre-Saturation/1 -> Clamping circuit/1(preSat)
  Post-Saturation/1 -> Clamping circuit/2(postSat)
  Clamping circuit/1(Clamp) -> Clamp Switch/2
  Constant/1 -> Clamp Switch/1
  Discrete-Time Integrator/1 -> Sum2/1
  POut/1 -> Sum2/2
  P/1 -> POut/2
  u/1 -> POut/1, IOut/2
  I/1 -> IOut/1

== system SkywalkerX8_GuidanceAndNavigation_Verification/Autopilot Digital/Gain Scheduled Controller Theta Digital/DF Controller Theta ==
  N : Inport
  D : Inport  Port=2
  du/dt : Inport  Port=3
  Discrete-Time Integrator : DiscreteIntegrator  SampleTime=SkywalkerX8.Control.Longitudinal.thetaController.Digital.SampleTime  ICPrevOutput=DiscIntNeverNeededParam  ICPrevScaledInput=DiscIntNeverNeededParam
  Product : Product
  Product1 : Product
  Sum : Sum  Inputs=|+-
  de* : Outport
  wires:
  Discrete-Time Integrator/1 -> de*/1, Sum/2  "de*"
  Product1/1 -> Discrete-Time Integrator/1  "Nde*_e"
  du/dt/1 -> Product/2
  D/1 -> Product/1
  Sum/1 -> Product1/2  "de*_e"
  N/1 -> Product1/1
  Product/1 -> Sum/1

== system SkywalkerX8_GuidanceAndNavigation_Verification/Autopilot Digital/Gain Scheduled Controller Theta Digital/PDF Controller Theta 2DOF ==
  u : Inport
  P : Inport  Port=2
  D : Inport  Port=3
  N : Inport  Port=4
  Discrete-Time Integrator : DiscreteIntegrator  InitialCondition=SkywalkerX8.InitialConditions.ThetaController.RefController.Derivative  SampleTime=SkywalkerX8.Control.Longitudinal.thetaController.Digital.SampleTime  ICPrevOutput=DiscIntNeverNeededParam  ICPrevScaledInput=DiscIntNeverNeededParam
  POut : Product
  Product : Product
  Product1 : Product
  Sum : Sum  Inputs=|+-
  Sum2 : Sum
  y : Outport  InitialOutput=0
  wires:
  Sum2/1 -> y/1
  N/1 -> Product1/1
  Product1/1 -> Discrete-Time Integrator/1, Sum2/2
  Sum/1 -> Product1/2
  POut/1 -> Sum2/1
  D/1 -> Product/2
  u/1 -> Product/1, POut/2  "u"
  Discrete-Time Integrator/1 -> Sum/2
  Product/1 -> Sum/1
  P/1 -> POut/1

== system SkywalkerX8_GuidanceAndNavigation_Verification/Autopilot Digital/Gain Scheduled Controller Theta Digital/PI Controller Theta ==
  u : Inport
  P : Inport  Port=2
  I : Inport  Port=3
  Post-Saturation : Inport  Port=4
  Pre-Saturation : Inport  Port=5
  Clamp Switch : Switch  Criteria=u2 ~= 0
  Clamping circuit : Subsystem
  Constant : Constant  Value=0
  Discrete-Time Integrator : DiscreteIntegrator  IntegratorMethod=Integration: Trapezoidal  InitialCondition=SkywalkerX8.InitialConditions.ThetaController.Integrator  SampleTime=SkywalkerX8.Control.Longitudinal.thetaController.Digital.SampleTime  ICPrevOutput=DiscIntNeverNeededParam  ICPrevScaledInput=DiscIntNeverNeededParam
  IOut : Product  DisableCoverage=on
  POut : Product
  Sum2 : Sum  Inputs=|++
  y : Outport  InitialOutput=0
  wires:
  IOut/1 -> Clamp Switch/3
  Clamp Switch/1 -> Discrete-Time Integrator/1
  Sum2/1 -> y/1
  Pre-Saturation/1 -> Clamping circuit/1(preSat)
  Post-Saturation/1 -> Clamping circuit/2(postSat)
  Clamping circuit/1(Clamp) -> Clamp Switch/2
  Constant/1 -> Clamp Switch/1
  Discrete-Time Integrator/1 -> Sum2/1
  POut/1 -> Sum2/2
  P/1 -> POut/2
  u/1 -> POut/1, IOut/2
  I/1 -> IOut/1

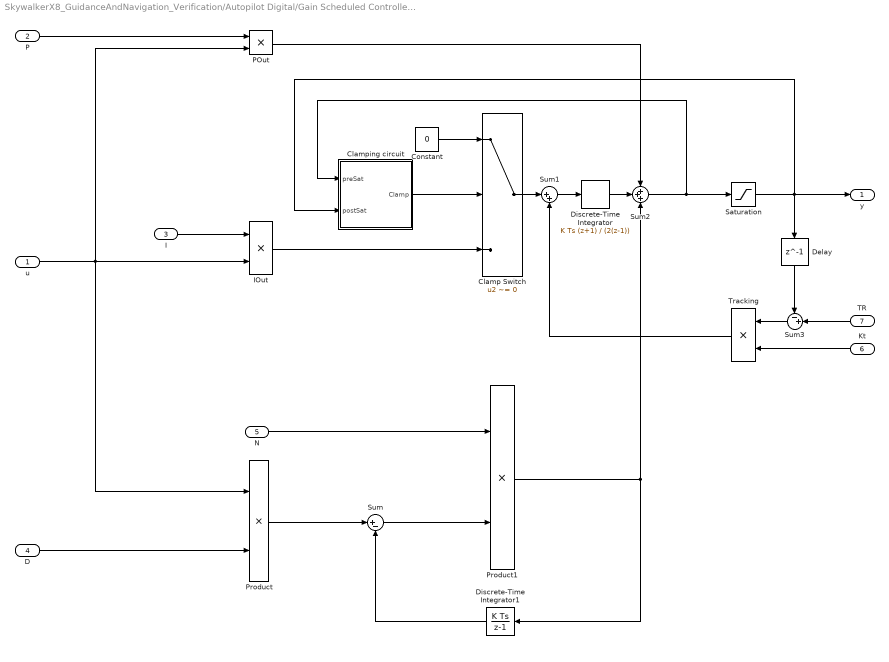
== system SkywalkerX8_GuidanceAndNavigation_Verification/Autopilot Digital/Gain Scheduled Controller Va_dt Digital/PIDF Controller Va_dt ==
  u : Inport
  P : Inport  Port=2
  I : Inport  Port=3
  D : Inport  Port=4
  N : Inport  Port=5
  Kt : Inport  Port=6
  TR : Inport  Port=7
  Clamp Switch : Switch  Criteria=u2 ~= 0
  Clamping circuit : Subsystem
  Constant : Constant  Value=0
  Delay : Delay  DelayLength=1  InitialCondition=SkywalkerX8.InitialConditions.dt
  Discrete-Time Integrator : DiscreteIntegrator  IntegratorMethod=Integration: Trapezoidal  InitialCondition=SkywalkerX8.InitialConditions.dt  SampleTime=SkywalkerX8.Control.Longitudinal.VaDtController.Digital.SampleTime  ICPrevOutput=DiscIntNeverNeededParam  ICPrevScaledInput=DiscIntNeverNeededParam
  Discrete-Time Integrator1 : DiscreteIntegrator  SampleTime=SkywalkerX8.Control.Longitudinal.VaDtController.Digital.SampleTime  ICPrevOutput=DiscIntNeverNeededParam  ICPrevScaledInput=DiscIntNeverNeededParam
  IOut : Product  DisableCoverage=on
  POut : Product
  Product : Product
  Product1 : Product
  Saturation : Saturate  UpperLimit=SkywalkerX8.Control.Longitudinal.VaDtController.upperSaturationDt  LowerLimit=SkywalkerX8.Control.Longitudinal.VaDtController.lowerSaturationDt
  Sum : Sum  Inputs=|+-
  Sum1 : Sum  Inputs=|++
  Sum2 : Sum  Inputs=+++
  Sum3 : Sum  Inputs=-+|
  Tracking : Product  DisableCoverage=on
  y : Outport  InitialOutput=0
  wires:
  Saturation/1 -> Clamping circuit/2(postSat), y/1, Delay/1
  N/1 -> Product1/1
  Product1/1 -> Discrete-Time Integrator1/1, Sum2/3
  Sum2/1 -> Saturation/1, Clamping circuit/1(preSat)
  Sum/1 -> Product1/2
  POut/1 -> Sum2/1
  D/1 -> Product/2
  u/1 -> Product/1, POut/2, IOut/2
  Discrete-Time Integrator1/1 -> Sum/2
  Clamp Switch/1 -> Sum1/1
  Product/1 -> Sum/1
  Discrete-Time Integrator/1 -> Sum2/2
  Constant/1 -> Clamp Switch/1
  I/1 -> IOut/1
  IOut/1 -> Clamp Switch/3
  Clamping circuit/1(Clamp) -> Clamp Switch/2
  P/1 -> POut/1
  TR/1 -> Sum3/2
  Sum3/1 -> Tracking/1
  Kt/1 -> Tracking/2
  Tracking/1 -> Sum1/2
  Sum1/1 -> Discrete-Time Integrator/1
  Delay/1 -> Sum3/1

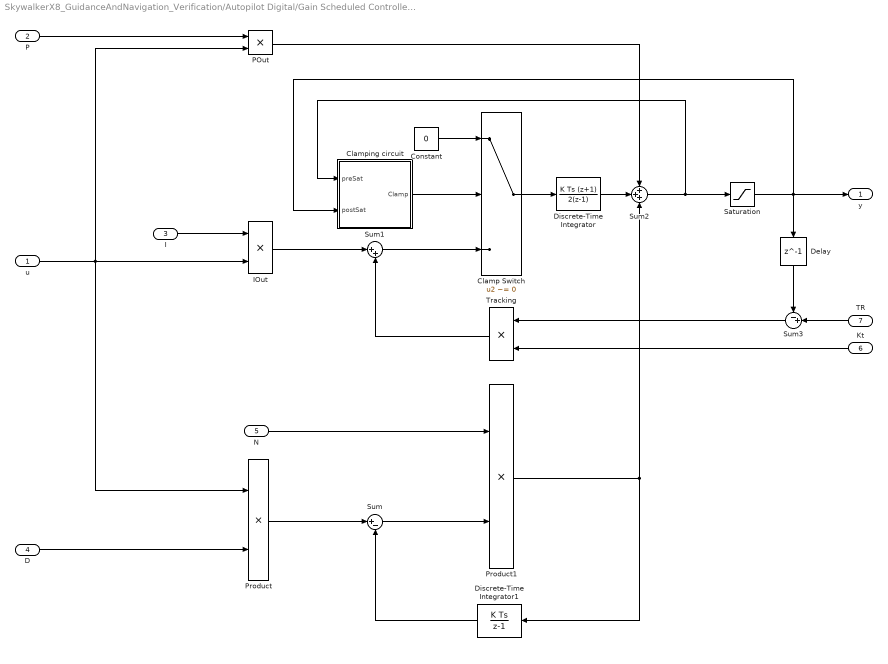
== system SkywalkerX8_GuidanceAndNavigation_Verification/Autopilot Digital/Gain Scheduled Controller Va_theta Digital/PIDF Controller Va_theta ==
  u : Inport
  P : Inport  Port=2
  I : Inport  Port=3
  D : Inport  Port=4
  N : Inport  Port=5
  Kt : Inport  Port=6
  TR : Inport  Port=7
  Clamp Switch : Switch  Criteria=u2 ~= 0
  Clamping circuit : Subsystem
  Constant : Constant  Value=0
  Delay : Delay  DelayLength=1  InitialCondition=-SkywalkerX8.InitialConditions.PhiThetaPsi(2)
  Discrete-Time Integrator : DiscreteIntegrator  IntegratorMethod=Integration: Trapezoidal  InitialCondition=-SkywalkerX8.InitialConditions.PhiThetaPsi(2)  SampleTime=SkywalkerX8.Control.Longitudinal.VaThetaController.Digital.SampleTime  ICPrevOutput=DiscIntNeverNeededParam  ICPrevScaledInput=DiscIntNeverNeededParam
  Discrete-Time Integrator1 : DiscreteIntegrator  SampleTime=SkywalkerX8.Control.Longitudinal.VaThetaController.Digital.SampleTime  ICPrevOutput=DiscIntNeverNeededParam  ICPrevScaledInput=DiscIntNeverNeededParam
  IOut : Product  DisableCoverage=on
  POut : Product
  Product : Product
  Product1 : Product
  Saturation : Saturate  UpperLimit=SkywalkerX8.Control.Longitudinal.VaThetaController.upperSaturationThetaC  LowerLimit=SkywalkerX8.Control.Longitudinal.VaThetaController.lowerSaturationThetaC
  Sum : Sum  Inputs=|+-
  Sum1 : Sum  Inputs=|++
  Sum2 : Sum  Inputs=+++
  Sum3 : Sum  Inputs=-+|
  Tracking : Product  DisableCoverage=on
  y : Outport  InitialOutput=0
  wires:
  Saturation/1 -> Clamping circuit/2(postSat), y/1, Delay/1
  N/1 -> Product1/1
  Product1/1 -> Discrete-Time Integrator1/1, Sum2/3
  Sum2/1 -> Saturation/1, Clamping circuit/1(preSat)
  Sum/1 -> Product1/2
  POut/1 -> Sum2/1
  D/1 -> Product/2
  u/1 -> Product/1, POut/2, IOut/2
  Discrete-Time Integrator1/1 -> Sum/2
  Clamp Switch/1 -> Discrete-Time Integrator/1
  Product/1 -> Sum/1
  Discrete-Time Integrator/1 -> Sum2/2
  Constant/1 -> Clamp Switch/1
  I/1 -> IOut/1
  Sum1/1 -> Clamp Switch/3
  Clamping circuit/1(Clamp) -> Clamp Switch/2
  P/1 -> POut/1
  IOut/1 -> Sum1/1
  TR/1 -> Sum3/2
  Sum3/1 -> Tracking/1
  Kt/1 -> Tracking/2
  Tracking/1 -> Sum1/2
  Delay/1 -> Sum3/1

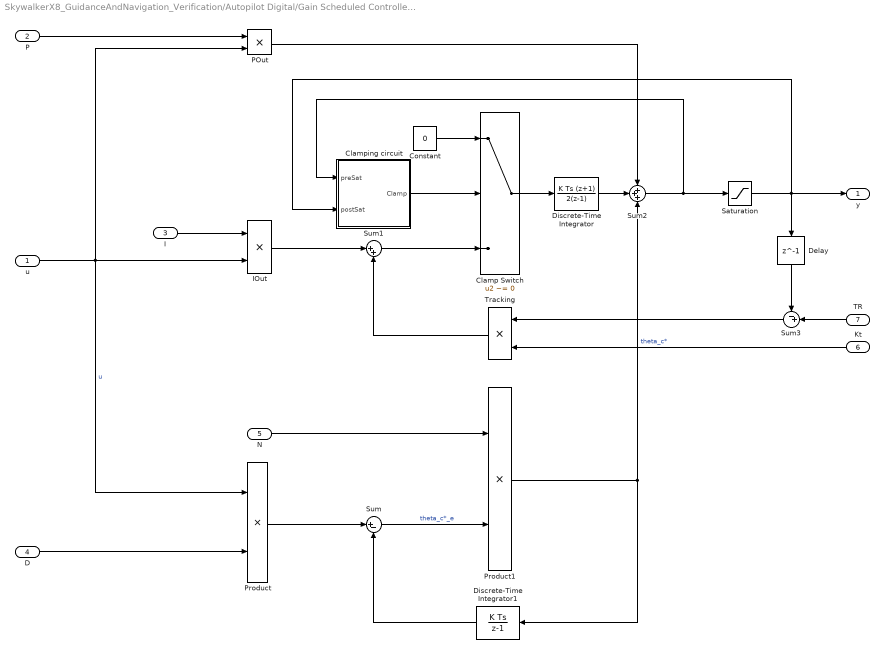
== system SkywalkerX8_GuidanceAndNavigation_Verification/Autopilot Digital/Gain Scheduled Controller h_theta Digital/PIDF Controller h_theta ==
  u : Inport
  P : Inport  Port=2
  I : Inport  Port=3
  D : Inport  Port=4
  N : Inport  Port=5
  Kt : Inport  Port=6
  TR : Inport  Port=7
  Clamp Switch : Switch  Criteria=u2 ~= 0
  Clamping circuit : Subsystem
  Constant : Constant  Value=0
  Delay : Delay  DelayLength=1  InitialCondition=SkywalkerX8.InitialConditions.PhiThetaPsi(2)
  Discrete-Time Integrator : DiscreteIntegrator  IntegratorMethod=Integration: Trapezoidal  InitialCondition=SkywalkerX8.InitialConditions.PhiThetaPsi(2)  SampleTime=SkywalkerX8.Control.Longitudinal.altController.Digital.SampleTime  ICPrevOutput=DiscIntNeverNeededParam  ICPrevScaledInput=DiscIntNeverNeededParam
  Discrete-Time Integrator1 : DiscreteIntegrator  SampleTime=SkywalkerX8.Control.Longitudinal.altController.Digital.SampleTime  ICPrevOutput=DiscIntNeverNeededParam  ICPrevScaledInput=DiscIntNeverNeededParam
  IOut : Product  DisableCoverage=on
  POut : Product
  Product : Product
  Product1 : Product
  Saturation : Saturate  UpperLimit=SkywalkerX8.Control.Longitudinal.altController.upperSaturationThetaC  LowerLimit=SkywalkerX8.Control.Longitudinal.altController.lowerSaturationThetaC
  Sum : Sum  Inputs=|+-
  Sum1 : Sum  Inputs=|++
  Sum2 : Sum  Inputs=+++
  Sum3 : Sum  Inputs=-+|
  Tracking : Product  DisableCoverage=on
  y : Outport  InitialOutput=0
  wires:
  Saturation/1 -> Clamping circuit/2(postSat), y/1, Delay/1
  Sum2/1 -> Saturation/1, Clamping circuit/1(preSat)
  POut/1 -> Sum2/1
  Clamp Switch/1 -> Discrete-Time Integrator/1
  Discrete-Time Integrator/1 -> Sum2/2
  Constant/1 -> Clamp Switch/1
  I/1 -> IOut/1
  Sum1/1 -> Clamp Switch/3
  Clamping circuit/1(Clamp) -> Clamp Switch/2
  P/1 -> POut/1
  IOut/1 -> Sum1/1
  TR/1 -> Sum3/2
  Sum3/1 -> Tracking/1
  Kt/1 -> Tracking/2
  Tracking/1 -> Sum1/2
  Discrete-Time Integrator1/1 -> Sum/2
  D/1 -> Product/2
  Product/1 -> Sum/1
  N/1 -> Product1/1
  Product1/1 -> Sum2/3, Discrete-Time Integrator1/1  "theta_c*"
  u/1 -> Product/1, POut/2, IOut/2  "u"
  Sum/1 -> Product1/2  "theta_c*_e"
  Delay/1 -> Sum3/1

== system SkywalkerX8_GuidanceAndNavigation_Verification/Guidance and Navigation/Path Following Algorithm/Straight Line//Orbit Following Selection ==
  Straight Line : Inport
  Flag : Inport  Port=2
  Orbit : Inport  Port=3
  Multiport Switch : MultiPortSwitch  Inputs=2  DiagnosticForDefault=Warning
  "[h_c, chi_c]" : Outport
  wires:
  Orbit/1 -> Multiport Switch/3
  Flag/1 -> Multiport Switch/1
  Straight Line/1 -> Multiport Switch/2
  Multiport Switch/1 -> "[h_c, chi_c]"/1
